simulink model "Part2_1"  (R2022a)
settings: Solver=VariableStepAuto  StartTime=0.0  StopTime=10  RelTol=1e-3
values from neighbouring files (symbols this model uses):
  D = diag([0.01, 0.01, 0.01])    [driver2.m]    (also in driver2_2.m; driver2_3.m; driver_2_2.m)
  g = [0,0,-9.81]    [driver2.m]    (also in driver2_2.m; driver2_3.m; driver_2_2.m)
  I = diag([3e-6, 3e-6, 1e-5])    [driver2.m]    (also in driver2_2.m; driver2_3.m; driver_2_2.m)
  In = inv(I)    [driver2.m]    (also in driver2_2.m; driver2_3.m; driver_2_2.m)
  k = 0.01    [driver2.m]    (also in driver2_2.m; driver2_3.m; driver_2_2.m)
  m = 0.5    [driver2.m]    (also in driver2_2.m; driver2_3.m; driver_2_2.m)
  omg_vec = [0 ... (first row only)    [driver2.m]    (also in driver2_2.m; driver2_3.m; driver_2_2.m)
  tau = [L*k*(Omega(1)^2 - Omega(3)^2) ... (first row only)    [driver2.m]    (also in driver2_2.m; driver2_3.m = 2*w0*[L*k*(Omega(1) - Omega(3)); driver_2_2.m)
libraries: matrix_library x1
settings Model: Creator=askeo  LastModifiedBy=askeo

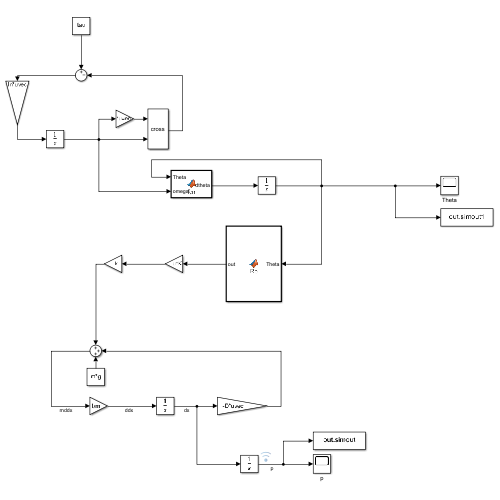
[thumbnail: Simulink's stored preview of the top-level diagram]
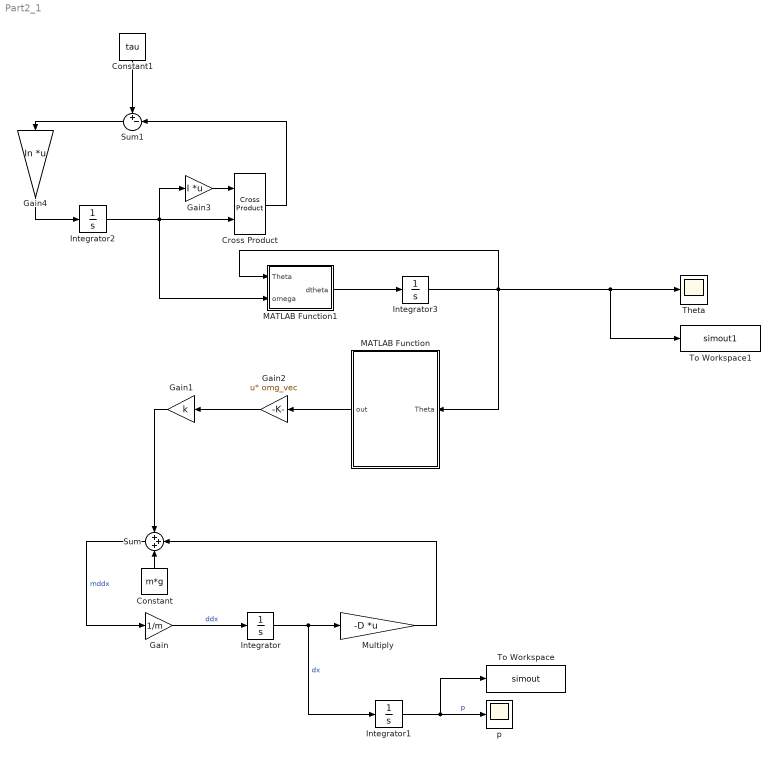
== system Part2_1 ==
  Constant : Constant  Value=m*g
  Constant1 : Constant  Value=tau
  Cross Product : matrix_library/Cross Product
      settings: SourceProductBaseCode=SL
  Gain : Gain  Gain=1/m
  Gain1 : Gain  Gain=k
  Gain2 : Gain  Gain=omg_vec  Multiplication=Matrix(u*K)
  Gain3 : Gain  Gain=I  Multiplication=Matrix(K*u) (u vector)
  Gain4 : Gain  Gain=In  Multiplication=Matrix(K*u) (u vector)
  Integrator : Integrator  InitialCondition=[0;0;0]
  Integrator1 : Integrator  InitialCondition=[0;0;0]
  Integrator2 : Integrator  InitialCondition=[0;0;0]
  Integrator3 : Integrator  InitialCondition=[0; 0; 0]
  MATLAB Function : MATLAB Function  TreatAsAtomicUnit=on
  MATLAB Function1 : MATLAB Function  TreatAsAtomicUnit=on
  Multiply : Gain  Gain=-D  Multiplication=Matrix(K*u) (u vector)
  Sum : Sum  Inputs=+++
  Sum1 : Sum  Inputs=+-|
  Theta : Scope
  To Workspace : ToWorkspace  VariableName=simout  SaveFormat=Timeseries  SampleTime=-1
  To Workspace1 : ToWorkspace  VariableName=simout1  SaveFormat=Timeseries  SampleTime=-1
  p : Scope
  wires:
  Gain/1 -> Integrator/1  "ddx"
  Integrator/1 -> Integrator1/1, Multiply/1  "dx"
  Multiply/1 -> Sum/2
  Constant/1 -> Sum/3
  Gain1/1 -> Sum/1
  Sum/1 -> Gain/1  "mddx"
  Integrator1/1 -> To Workspace/1, p/1  "p"
  Integrator2/1 -> MATLAB Function1/2(omega), Gain3/1, Cross Product/2
  MATLAB Function1/1(dtheta) -> Integrator3/1
  MATLAB Function/1(out) -> Gain2/1
  Constant1/1 -> Sum1/1
  Cross Product/1 -> Sum1/2
  Sum1/1 -> Gain4/1
  Gain4/1 -> Integrator2/1
  Gain3/1 -> Cross Product/1
  Gain2/1 -> Gain1/1
  Integrator3/1 -> MATLAB Function1/1(Theta), MATLAB Function/1(Theta), To Workspace1/1, Theta/1

== matlab function Part2_1/MATLAB Function1 ==
  data: dtheta output; Theta input; omega input
function dtheta = fcn(Theta, omega)

C = [1, 0, -sin(Theta(2))
    0, cos(Theta(1)), cos(Theta(2))*sin(Theta(1))
    0, -sin(Theta(1)), cos(Theta(2))*cos(Theta(1))];

dtheta = inv(C)*omega;
end

== matlab function Part2_1/MATLAB Function ==
  data: Theta input; out output
function out = Rb(Theta)

phi = Theta(1);
theta = Theta(2);
psi = Theta(3);

rbi = [cos(psi)*cos(theta), cos(psi)*sin(theta)*sin(phi) - sin(psi)*cos(phi), sin(psi)*sin(phi) + cos(psi)*sin(theta)*cos(phi)
    sin(psi)*cos(theta), cos(psi)*cos(phi) + sin(psi)*sin(theta)*sin(phi), sin(psi)*sin(theta)*sin(phi) - cos(psi)*sin(phi)
    -sin(theta), cos(theta)*sin(phi), cos(theta)*cos(phi)];

out = rbi;
end
